simulink model "ALL_JP360_DBW_V6_5_1103"  (R2022a)
settings: Solver=FixedStepAuto  StartTime=0.0  StopTime=inf  FixedStep=0.01  RelTol=1e-3  EnableMultiTasking=on
model workspace (MAT data in the model file):
  g = 9.8
undefined symbols (not defined in the file or in its folder): canChannel, delta_v_p, IPM_Line_C0, IPM_Line_C1, IPM_Line_C2, IPM_Line_C3, M, M_p, MRR_ObjDistX, MRR_ObjDistY, MRR_ObjFusionCamID, MRR_ObjFusionSig, MRR_ObjID, MRR_ObjRelVelX, MRR_ObjRelVelY, MRR_ObjType, MRR_ObjUpdFlg, none, obj_vaild, untracktime, V, videoinput
libraries: canfdmsglib x230, canfdlib x76, slpidlib x24, simulink x18, dspstat3 x14, ctrlSharedLib x1, simulink_extras x1, imaqlib x1, realtime_pacer_lib x1, dspvision x1, visionsinks x1
(part 29 of 55)

== system ALL_JP360_DBW_V6_5_1103/MsgFromCAN/SRR_ADCU_MsgFromCAN/SRR_ADCU_RLR_Freespace_0x1F4 ==
  SRR_ADCU_RLR_Freespace_0x1F4FromInData : Inport  OutDataTypeStr=Bus:CAN_FD_MESSAGE_BUS
  Bus Creator : BusCreator  Inputs=56  OutDataTypeStr=Bus:SRR_ADCU_RLR_Freespace_0x1F4  NonVirtualBus=on
  CAN FD Unpack : canfdmsglib/CAN FD Unpack  CANdbFile=V363 SRR Private CAN-V1.3.dbc  MsgList=(none)  MsgName=RLR_Freespace_0x1F4  ProtocolMode=CAN FD  MsgIDType=Standard (11-bit identifier)  MsgIdentifier=500  MsgLength=64  SignalInfo={'RLR_CRCCheck_FSP_MSG4','504','16','BE','unsigned','Standard','0','1','0','0','65535';'RLR_FreespaceSectorConfidence103','12','2','BE','unsigned','Standard','0','1','0','0','3';'RLR_FreespaceSectorConfidence104','30','2','BE','unsigned','Standard','0','1','0','0','3';'RLR_FreespaceSectorConfidence105','32','2','BE','unsigned','Standard','0','1','0','0','3';'RLR_FreespaceSectorConfidence106','50','2','BE','unsigned','Standard','0','1','0','0','3';'RLR_FreespaceSectorConfidence107','68','2','BE','unsigned','Standard','0','1','0','0','3';'RLR_FreespaceSectorConfidence108','86','2','BE','unsigned','Standard','0','1','0','0','3';'RLR_FreespaceSectorConfidence109','88','2','BE','unsigned','Standard','0','1','0','0','3';'RLR_FreespaceSectorConfidence110','106','2','BE','unsigned','Standard','0','1','0','0','3';'RLR_FreespaceSectorConfidence111','124','2','BE','unsigned','Standard','0','1','0','0','3';'RLR_FreespaceSectorConfidence112','142','2','BE','unsigned','Standard','0','1','0','0','3';'RLR_FreespaceSectorConfidence113','144','2','BE','unsigned','Standard','0','1','0','0','3';'RLR_FreespaceSectorConfidence114','162','2','BE','unsigned','Standard','0','1','0','0','3';'RLR_FreespaceSectorConfidence115','180','2','BE','unsigned','Standard','0','1','0','0','3';'RLR_FreespaceSectorConfidence116','198','2','BE','unsigned','Standard','0','1','0','0','3';'RLR_FreespaceSectorConfidence117','200','2','BE','unsigned','Standard','0','1','0','0','3';'RLR_FreespaceSectorConfidence118','218','2','BE','unsigned','Standard','0','1','0','0','3';'RLR_FreespaceSectorConfidence119','236','2','BE','unsigned','Standard','0','1','0','0','3';'RLR_FreespaceSectorConfidence120','254','2','BE','unsigned','Standard','0','1','0','0','3';'RLR_FreespaceSectorDistance103','14','10','BE','unsigned','Standard','0','0.1','0','0','100';'RLR_FreespaceSectorDistance104','16','10','BE','unsigned','Standard','0','0.1','0','0','100';'RLR_FreespaceSectorDistance105','34','10','BE','unsigned','Standard','0','0.1','0','0','100';'RLR_FreespaceSectorDistance106','52','10','BE','unsigned','Standard','0','0.1','0','0','100';'RLR_FreespaceSectorDistance107','70','10','BE','unsigned','Standard','0','0.1','0','0','100';'RLR_FreespaceSectorDistance108','72','10','BE','unsigned','Standard','0','0.1','0','0','100';'RLR_FreespaceSectorDistance109','90','10','BE','unsigned','Standard','0','0.1','0','0','100';'RLR_FreespaceSectorDistance110','108','10','BE','unsigned','Standard','0','0.1','0','0','100';'RLR_FreespaceSectorDistance111','126','10','BE','unsigned','Standard','0','0.1','0','0','100';'RLR_FreespaceSectorDistance112','128','10','BE','unsigned','Standard','0','0.1','0','0','100';'RLR_FreespaceSectorDistance113','146','10','BE','unsigned','Standard','0','0.1','0','0','100';'RLR_FreespaceSectorDistance114','164','10','BE','unsigned','Standard','0','0.1','0','0','100';'RLR_FreespaceSectorDistance115','182','10','BE','unsigned','Standard','0','0.1','0','0','100';'RLR_FreespaceSectorDistance116','184','10','BE','unsigned','Standard','0','0.1','0','0','100';'RLR_FreespaceSectorDistance117','202','10','BE','unsigned','Standard','0','0.1','0','0','100';'RLR_FreespaceSectorDistance118','220','10','BE','unsigned','Standard','0','0.1','0','0','100';'RLR_FreespaceSectorDistance119','238','10','BE','unsigned','Standard','0','0.1','0','0','100';'RLR_FreespaceSectorDistance120','240','10','BE','unsigned','Standard','0','0.1','0','0','100';'RLR_FreespaceSectorKinestate103','10','2','BE','unsigned','Standard','0','1','0','0','3';'RLR_FreespaceSectorKinestate104','28','2','BE','unsigned','Standard','0','1','0','0','3';'RLR_FreespaceSectorKinestate105','46','2','BE','unsigned','Standard','0','1','0','0','3';'RLR_FreespaceSectorKinestate106','48','2','BE','unsigned','Standard','0','1','0','0','3';'RLR_FreespaceSectorKinestate107','66','2','BE','unsigned','Standard','0','1','0','0','3';'RLR_FreespaceSectorKinestate108','84','2','BE','unsigned','Standard','0','1','0','0','3';'RLR_FreespaceSectorKinestate109','102','2','BE','unsigned','Standard','0','1','0','0','3';'RLR_FreespaceSectorKinestate110','104','2','BE','unsigned','Standard','0','1','0','0','3';'RLR_FreespaceSectorKinestate111','122','2','BE','unsigned','Standard','0','1','0','0','3';'RLR_FreespaceSectorKinestate112','140','2','BE','unsigned','Standard','0','1','0','0','3';'RLR_FreespaceSectorKinestate113','158','2','BE','unsigned','Standard','0','1','0','0','3';'RLR_FreespaceSectorKinestate114','160','2','BE','unsigned','Standard','0','1','0','0','3';'RLR_FreespaceSectorKinestate115','178','2','BE','unsigned','Standard','0','1','0','0','3';'RLR_FreespaceSectorKinestate116','196','2','BE','unsigned','Standard','0','1','0','0','3';'RLR_FreespaceSectorKinestate117','214','2','BE','unsigned','Standard','0','1','0','0','3';'RLR_FreespaceSectorKinestate118','216','2','BE','unsigned','Standard','0','1','0','0','3';'RLR_FreespaceSectorKinestate119','234','2','BE','unsigned','Standard','0','1','0','0','3';'RLR_FreespaceSectorKinestate120','252','2','BE','unsigned','Standard','0','1','0','0','3';'RLR_RollingCounter_FSP_MSG4','488','4','BE','unsigned','Standard','0','1','0','0','15'}  IDPort=off  TimestampPort=off  ErrorPort=off  RemotePort=off  LengthPort=off  StatusPort=off  BRSPort=off  ESIPort=off  DLCPort=off  ApplyMinMax=off
      settings: SourceProductBaseCode=ME,XP,VN  DataFormat=CANdb specified signals
  Data Type Conversion1 : DataTypeConversion  OutDataTypeStr=uint16  SaturateOnIntegerOverflow=off  RndMeth=Floor
  Data Type Conversion{2..19,38..56} (37 alike) : DataTypeConversion  OutDataTypeStr=int8  SaturateOnIntegerOverflow=off  RndMeth=Floor
  Data Type Conversion{20..37} (18 alike) : DataTypeConversion  OutDataTypeStr=single  SaturateOnIntegerOverflow=off  RndMeth=Floor
  SRR_ADCU_RLR_Freespace_0x1F4FromOutData : Outport  OutDataTypeStr=Bus:SRR_ADCU_RLR_Freespace_0x1F4
  wires:
  CAN FD Unpack/1 -> Data Type Conversion1/1
  CAN FD Unpack/2 -> Data Type Conversion2/1
  CAN FD Unpack/3 -> Data Type Conversion3/1
  CAN FD Unpack/4 -> Data Type Conversion4/1
  CAN FD Unpack/5 -> Data Type Conversion5/1
  CAN FD Unpack/6 -> Data Type Conversion6/1
  CAN FD Unpack/7 -> Data Type Conversion7/1
  CAN FD Unpack/8 -> Data Type Conversion8/1
  CAN FD Unpack/9 -> Data Type Conversion9/1
  CAN FD Unpack/10 -> Data Type Conversion10/1
  CAN FD Unpack/11 -> Data Type Conversion11/1
  CAN FD Unpack/12 -> Data Type Conversion12/1
  CAN FD Unpack/13 -> Data Type Conversion13/1
  CAN FD Unpack/14 -> Data Type Conversion14/1
  CAN FD Unpack/15 -> Data Type Conversion15/1
  CAN FD Unpack/16 -> Data Type Conversion16/1
  CAN FD Unpack/17 -> Data Type Conversion17/1
  CAN FD Unpack/18 -> Data Type Conversion18/1
  CAN FD Unpack/19 -> Data Type Conversion19/1
  CAN FD Unpack/20 -> Data Type Conversion20/1
  CAN FD Unpack/21 -> Data Type Conversion21/1
  CAN FD Unpack/22 -> Data Type Conversion22/1
  CAN FD Unpack/23 -> Data Type Conversion23/1
  CAN FD Unpack/24 -> Data Type Conversion24/1
  CAN FD Unpack/25 -> Data Type Conversion25/1
  CAN FD Unpack/26 -> Data Type Conversion26/1
  CAN FD Unpack/27 -> Data Type Conversion27/1
  CAN FD Unpack/28 -> Data Type Conversion28/1
  CAN FD Unpack/29 -> Data Type Conversion29/1
  CAN FD Unpack/30 -> Data Type Conversion30/1
  CAN FD Unpack/31 -> Data Type Conversion31/1
  CAN FD Unpack/32 -> Data Type Conversion32/1
  CAN FD Unpack/33 -> Data Type Conversion33/1
  CAN FD Unpack/34 -> Data Type Conversion34/1
  CAN FD Unpack/35 -> Data Type Conversion35/1
  CAN FD Unpack/36 -> Data Type Conversion36/1
  CAN FD Unpack/37 -> Data Type Conversion37/1
  CAN FD Unpack/38 -> Data Type Conversion38/1
  CAN FD Unpack/39 -> Data Type Conversion39/1
  CAN FD Unpack/40 -> Data Type Conversion40/1
  CAN FD Unpack/41 -> Data Type Conversion41/1
  CAN FD Unpack/42 -> Data Type Conversion42/1
  CAN FD Unpack/43 -> Data Type Conversion43/1
  CAN FD Unpack/44 -> Data Type Conversion44/1
  CAN FD Unpack/45 -> Data Type Conversion45/1
  CAN FD Unpack/46 -> Data Type Conversion46/1
  CAN FD Unpack/47 -> Data Type Conversion47/1
  CAN FD Unpack/48 -> Data Type Conversion48/1
  CAN FD Unpack/49 -> Data Type Conversion49/1
  CAN FD Unpack/50 -> Data Type Conversion50/1
  CAN FD Unpack/51 -> Data Type Conversion51/1
  CAN FD Unpack/52 -> Data Type Conversion52/1
  CAN FD Unpack/53 -> Data Type Conversion53/1
  CAN FD Unpack/54 -> Data Type Conversion54/1
  CAN FD Unpack/55 -> Data Type Conversion55/1
  CAN FD Unpack/56 -> Data Type Conversion56/1
  Data Type Conversion1/1 -> Bus Creator/1  "RLR_CRCCheck_FSP_MSG4"
  Data Type Conversion2/1 -> Bus Creator/2  "RLR_FreespaceSectorConfidence103"
  Data Type Conversion3/1 -> Bus Creator/3  "RLR_FreespaceSectorConfidence104"
  Data Type Conversion4/1 -> Bus Creator/4  "RLR_FreespaceSectorConfidence105"
  Data Type Conversion5/1 -> Bus Creator/5  "RLR_FreespaceSectorConfidence106"
  Data Type Conversion6/1 -> Bus Creator/6  "RLR_FreespaceSectorConfidence107"
  Data Type Conversion7/1 -> Bus Creator/7  "RLR_FreespaceSectorConfidence108"
  Data Type Conversion8/1 -> Bus Creator/8  "RLR_FreespaceSectorConfidence109"
  Data Type Conversion9/1 -> Bus Creator/9  "RLR_FreespaceSectorConfidence110"
  Data Type Conversion10/1 -> Bus Creator/10  "RLR_FreespaceSectorConfidence111"
  Data Type Conversion11/1 -> Bus Creator/11  "RLR_FreespaceSectorConfidence112"
  Data Type Conversion12/1 -> Bus Creator/12  "RLR_FreespaceSectorConfidence113"
  Data Type Conversion13/1 -> Bus Creator/13  "RLR_FreespaceSectorConfidence114"
  Data Type Conversion14/1 -> Bus Creator/14  "RLR_FreespaceSectorConfidence115"
  Data Type Conversion15/1 -> Bus Creator/15  "RLR_FreespaceSectorConfidence116"
  Data Type Conversion16/1 -> Bus Creator/16  "RLR_FreespaceSectorConfidence117"
  Data Type Conversion17/1 -> Bus Creator/17  "RLR_FreespaceSectorConfidence118"
  Data Type Conversion18/1 -> Bus Creator/18  "RLR_FreespaceSectorConfidence119"
  Data Type Conversion19/1 -> Bus Creator/19  "RLR_FreespaceSectorConfidence120"
  Data Type Conversion20/1 -> Bus Creator/20  "RLR_FreespaceSectorDistance103"
  Data Type Conversion21/1 -> Bus Creator/21  "RLR_FreespaceSectorDistance104"
  Data Type Conversion22/1 -> Bus Creator/22  "RLR_FreespaceSectorDistance105"
  Data Type Conversion23/1 -> Bus Creator/23  "RLR_FreespaceSectorDistance106"
  Data Type Conversion24/1 -> Bus Creator/24  "RLR_FreespaceSectorDistance107"
  Data Type Conversion25/1 -> Bus Creator/25  "RLR_FreespaceSectorDistance108"
  Data Type Conversion26/1 -> Bus Creator/26  "RLR_FreespaceSectorDistance109"
  Data Type Conversion27/1 -> Bus Creator/27  "RLR_FreespaceSectorDistance110"
  Data Type Conversion28/1 -> Bus Creator/28  "RLR_FreespaceSectorDistance111"
  Data Type Conversion29/1 -> Bus Creator/29  "RLR_FreespaceSectorDistance112"
  Data Type Conversion30/1 -> Bus Creator/30  "RLR_FreespaceSectorDistance113"
  Data Type Conversion31/1 -> Bus Creator/31  "RLR_FreespaceSectorDistance114"
  Data Type Conversion32/1 -> Bus Creator/32  "RLR_FreespaceSectorDistance115"
  Data Type Conversion33/1 -> Bus Creator/33  "RLR_FreespaceSectorDistance116"
  Data Type Conversion34/1 -> Bus Creator/34  "RLR_FreespaceSectorDistance117"
  Data Type Conversion35/1 -> Bus Creator/35  "RLR_FreespaceSectorDistance118"
  Data Type Conversion36/1 -> Bus Creator/36  "RLR_FreespaceSectorDistance119"
  Data Type Conversion37/1 -> Bus Creator/37  "RLR_FreespaceSectorDistance120"
  Data Type Conversion38/1 -> Bus Creator/38  "RLR_FreespaceSectorKinestate103"
  Data Type Conversion39/1 -> Bus Creator/39  "RLR_FreespaceSectorKinestate104"
  Data Type Conversion40/1 -> Bus Creator/40  "RLR_FreespaceSectorKinestate105"
  Data Type Conversion41/1 -> Bus Creator/41  "RLR_FreespaceSectorKinestate106"
  Data Type Conversion42/1 -> Bus Creator/42  "RLR_FreespaceSectorKinestate107"
  Data Type Conversion43/1 -> Bus Creator/43  "RLR_FreespaceSectorKinestate108"
  Data Type Conversion44/1 -> Bus Creator/44  "RLR_FreespaceSectorKinestate109"
  Data Type Conversion45/1 -> Bus Creator/45  "RLR_FreespaceSectorKinestate110"
  Data Type Conversion46/1 -> Bus Creator/46  "RLR_FreespaceSectorKinestate111"
  Data Type Conversion47/1 -> Bus Creator/47  "RLR_FreespaceSectorKinestate112"
  Data Type Conversion48/1 -> Bus Creator/48  "RLR_FreespaceSectorKinestate113"
  Data Type Conversion49/1 -> Bus Creator/49  "RLR_FreespaceSectorKinestate114"
  Data Type Conversion50/1 -> Bus Creator/50  "RLR_FreespaceSectorKinestate115"
  Data Type Conversion51/1 -> Bus Creator/51  "RLR_FreespaceSectorKinestate116"
  Data Type Conversion52/1 -> Bus Creator/52  "RLR_FreespaceSectorKinestate117"
  Data Type Conversion53/1 -> Bus Creator/53  "RLR_FreespaceSectorKinestate118"
  Data Type Conversion54/1 -> Bus Creator/54  "RLR_FreespaceSectorKinestate119"
  Data Type Conversion55/1 -> Bus Creator/55  "RLR_FreespaceSectorKinestate120"
  Data Type Conversion56/1 -> Bus Creator/56  "RLR_RollingCounter_FSP_MSG4"
  Bus Creator/1 -> SRR_ADCU_RLR_Freespace_0x1F4FromOutData/1  "SRR_ADCU_RLR_Freespace_0x1F4FromOutData"
  SRR_ADCU_RLR_Freespace_0x1F4FromInData/1 -> CAN FD Unpack/1  "SRR_ADCU_RLR_Freespace_0x1F4FromInData"

== system ALL_JP360_DBW_V6_5_1103/MsgFromCAN/SRR_ADCU_MsgFromCAN/SRR_ADCU_RLR_OBJPos10_0x1CD ==
  SRR_ADCU_RLR_OBJPos10_0x1CDFromInData : Inport  OutDataTypeStr=Bus:CAN_FD_MESSAGE_BUS
  Bus Creator : BusCreator  Inputs=42  OutDataTypeStr=Bus:SRR_ADCU_RLR_OBJPos10_0x1CD  NonVirtualBus=on
  CAN FD Unpack : canfdmsglib/CAN FD Unpack  CANdbFile=V363 SRR Private CAN-V1.3.dbc  MsgList=(none)  MsgName=RLR_OBJPos10_0x1CD  ProtocolMode=CAN FD  MsgIDType=Standard (11-bit identifier)  MsgIdentifier=461  MsgLength=48  SignalInfo={'RLR_CRCCheck_0x1CD','376','16','BE','unsigned','Standard','0','1','0','0','65535';'RLR_OBJ19_Dx','79','13','BE','unsigned','Standard','0','0.0625','-256','-256','255.938';'RLR_OBJ19_Dy','60','11','BE','unsigned','Standard','0','0.125','-128','-128','127.875';'RLR_OBJ19_ExistProb','112','6','BE','unsigned','Standard','0','2','0','0','100';'RLR_OBJ19_HeadingAngle','55','10','BE','unsigned','Standard','0','0.01','-3.14','-3.14','3.14';'RLR_OBJ19_Height','26','9','BE','unsigned','Standard','0','0.01','0','0','5.11';'RLR_OBJ19_Length','33','9','BE','unsigned','Standard','0','0.05','0','0','25.5';'RLR_OBJ19_Measured','126','2','BE','unsigned','Standard','0','1','0','0','3';'RLR_OBJ19_Motion_Status','162','3','BE','unsigned','Standard','0','1','0','0','7';'RLR_OBJ19_ObstacleProb','120','6','BE','unsigned','Standard','0','2','0','0','100';'RLR_OBJ19_RefPointDx','144','13','BE','unsigned','Standard','0','0.0625','-256','-256','255.938';'RLR_OBJ19_RefPointDy','141','11','BE','unsigned','Standard','0','0.125','-128','-128','127.875';'RLR_OBJ19_RefPointLoc','157','3','BE','unsigned','Standard','0','1','0','0','7';'RLR_OBJ19_RelAx','118','9','BE','unsigned','Standard','0','0.0625','-16','-16','15.9375';'RLR_OBJ19_RelAy','111','10','BE','unsigned','Standard','0','0.03125','-16','-16','15.9688';'RLR_OBJ19_RelVx','89','12','BE','unsigned','Standard','0','0.0625','-128','-128','127.938';'RLR_OBJ19_RelVy','85','10','BE','unsigned','Standard','0','0.125','-64','-64','63.875';'RLR_OBJ19_Track_Age','165','8','BE','unsigned','Standard','0','1','0','0','255';'RLR_OBJ19_Track_ID','1','7','BE','unsigned','Standard','0','1','0','0','127';'RLR_OBJ19_Type','14','3','BE','unsigned','Standard','0','1','0','0','7';'RLR_OBJ19_Width','19','11','BE','unsigned','Standard','0','0.01','0','0','12';'RLR_OBJ20_Dx','247','13','BE','unsigned','Standard','0','0.0625','-256','-256','255.938';'RLR_OBJ20_Dy','228','11','BE','unsigned','Standard','0','0.125','-128','-128','127.875';'RLR_OBJ20_ExistProb','280','6','BE','unsigned','Standard','0','2','0','0','100';'RLR_OBJ20_HeadingAngle','223','10','BE','unsigned','Standard','0','0.01','-3.14','-3.14','3.14';'RLR_OBJ20_Height','194','9','BE','unsigned','Standard','0','0.01','0','0','5.11';'RLR_OBJ20_Length','201','9','BE','unsigned','Standard','0','0.05','0','0','25.5';'RLR_OBJ20_Measured','294','2','BE','unsigned','Standard','0','1','0','0','3';'RLR_OBJ20_Motion_Status','330','3','BE','unsigned','Standard','0','1','0','0','7';'RLR_OBJ20_ObstacleProb','288','6','BE','unsigned','Standard','0','2','0','0','100';'RLR_OBJ20_RefPointDx','312','13','BE','unsigned','Standard','0','0.0625','-256','-256','255.938';'RLR_OBJ20_RefPointDy','309','11','BE','unsigned','Standard','0','0.125','-128','-128','127.875';'RLR_OBJ20_RefPointLoc','325','3','BE','unsigned','Standard','0','1','0','0','7';'RLR_OBJ20_RelAx','286','9','BE','unsigned','Standard','0','0.0625','-16','-16','15.9375';'RLR_OBJ20_RelAy','279','10','BE','unsigned','Standard','0','0.03125','-16','-16','15.9688';'RLR_OBJ20_RelVx','257','12','BE','unsigned','Standard','0','0.0625','-128','-128','127.938';'RLR_OBJ20_RelVy','253','10','BE','unsigned','Standard','0','0.125','-64','-64','63.875';'RLR_OBJ20_Track_Age','333','8','BE','unsigned','Standard','0','1','0','0','255';'RLR_OBJ20_Track_ID','169','7','BE','unsigned','Standard','0','1','0','0','127';'RLR_OBJ20_Type','182','3','BE','unsigned','Standard','0','1','0','0','7';'RLR_OBJ20_Width','187','11','BE','unsigned','Standard','0','0.01','0','0','12';'RLR_RollingCounter_0x1CD','360','4','BE','unsigned','Standard','0','1','0','0','15'}  IDPort=off  TimestampPort=off  ErrorPort=off  RemotePort=off  LengthPort=off  StatusPort=off  BRSPort=off  ESIPort=off  DLCPort=off  ApplyMinMax=off
      settings: SourceProductBaseCode=ME,XP,VN  DataFormat=CANdb specified signals
  Data Type Conversion1 : DataTypeConversion  OutDataTypeStr=uint16  SaturateOnIntegerOverflow=off  RndMeth=Floor
  Data Type Conversion{4,8..10,13,19..20,24,28..30,33,39..40,42} (15 alike) : DataTypeConversion  OutDataTypeStr=int8  SaturateOnIntegerOverflow=off  RndMeth=Floor
  Data Type Conversion{2..3,5..7,11..12,14..17,21..23,25..27,31..32,34..37,41} (24 alike) : DataTypeConversion  OutDataTypeStr=single  SaturateOnIntegerOverflow=off  RndMeth=Floor
  Data Type Conversion18 : DataTypeConversion  OutDataTypeStr=uint8  SaturateOnIntegerOverflow=off  RndMeth=Floor
  Data Type Conversion38 : DataTypeConversion  OutDataTypeStr=uint8  SaturateOnIntegerOverflow=off  RndMeth=Floor
  SRR_ADCU_RLR_OBJPos10_0x1CDFromOutData : Outport  OutDataTypeStr=Bus:SRR_ADCU_RLR_OBJPos10_0x1CD
  wires:
  CAN FD Unpack/1 -> Data Type Conversion1/1
  CAN FD Unpack/2 -> Data Type Conversion2/1
  CAN FD Unpack/3 -> Data Type Conversion3/1
  CAN FD Unpack/4 -> Data Type Conversion4/1
  CAN FD Unpack/5 -> Data Type Conversion5/1
  CAN FD Unpack/6 -> Data Type Conversion6/1
  CAN FD Unpack/7 -> Data Type Conversion7/1
  CAN FD Unpack/8 -> Data Type Conversion8/1
  CAN FD Unpack/9 -> Data Type Conversion9/1
  CAN FD Unpack/10 -> Data Type Conversion10/1
  CAN FD Unpack/11 -> Data Type Conversion11/1
  CAN FD Unpack/12 -> Data Type Conversion12/1
  CAN FD Unpack/13 -> Data Type Conversion13/1
  CAN FD Unpack/14 -> Data Type Conversion14/1
  CAN FD Unpack/15 -> Data Type Conversion15/1
  CAN FD Unpack/16 -> Data Type Conversion16/1
  CAN FD Unpack/17 -> Data Type Conversion17/1
  CAN FD Unpack/18 -> Data Type Conversion18/1
  CAN FD Unpack/19 -> Data Type Conversion19/1
  CAN FD Unpack/20 -> Data Type Conversion20/1
  CAN FD Unpack/21 -> Data Type Conversion21/1
  CAN FD Unpack/22 -> Data Type Conversion22/1
  CAN FD Unpack/23 -> Data Type Conversion23/1
  CAN FD Unpack/24 -> Data Type Conversion24/1
  CAN FD Unpack/25 -> Data Type Conversion25/1
  CAN FD Unpack/26 -> Data Type Conversion26/1
  CAN FD Unpack/27 -> Data Type Conversion27/1
  CAN FD Unpack/28 -> Data Type Conversion28/1
  CAN FD Unpack/29 -> Data Type Conversion29/1
  CAN FD Unpack/30 -> Data Type Conversion30/1
  CAN FD Unpack/31 -> Data Type Conversion31/1
  CAN FD Unpack/32 -> Data Type Conversion32/1
  CAN FD Unpack/33 -> Data Type Conversion33/1
  CAN FD Unpack/34 -> Data Type Conversion34/1
  CAN FD Unpack/35 -> Data Type Conversion35/1
  CAN FD Unpack/36 -> Data Type Conversion36/1
  CAN FD Unpack/37 -> Data Type Conversion37/1
  CAN FD Unpack/38 -> Data Type Conversion38/1
  CAN FD Unpack/39 -> Data Type Conversion39/1
  CAN FD Unpack/40 -> Data Type Conversion40/1
  CAN FD Unpack/41 -> Data Type Conversion41/1
  CAN FD Unpack/42 -> Data Type Conversion42/1
  Data Type Conversion1/1 -> Bus Creator/1  "RLR_CRCCheck_0x1CD"
  Data Type Conversion2/1 -> Bus Creator/2  "RLR_OBJ19_Dx"
  Data Type Conversion3/1 -> Bus Creator/3  "RLR_OBJ19_Dy"
  Data Type Conversion4/1 -> Bus Creator/4  "RLR_OBJ19_ExistProb"
  Data Type Conversion5/1 -> Bus Creator/5  "RLR_OBJ19_HeadingAngle"
  Data Type Conversion6/1 -> Bus Creator/6  "RLR_OBJ19_Height"
  Data Type Conversion7/1 -> Bus Creator/7  "RLR_OBJ19_Length"
  Data Type Conversion8/1 -> Bus Creator/8  "RLR_OBJ19_Measured"
  Data Type Conversion9/1 -> Bus Creator/9  "RLR_OBJ19_Motion_Status"
  Data Type Conversion10/1 -> Bus Creator/10  "RLR_OBJ19_ObstacleProb"
  Data Type Conversion11/1 -> Bus Creator/11  "RLR_OBJ19_RefPointDx"
  Data Type Conversion12/1 -> Bus Creator/12  "RLR_OBJ19_RefPointDy"
  Data Type Conversion13/1 -> Bus Creator/13  "RLR_OBJ19_RefPointLoc"
  Data Type Conversion14/1 -> Bus Creator/14  "RLR_OBJ19_RelAx"
  Data Type Conversion15/1 -> Bus Creator/15  "RLR_OBJ19_RelAy"
  Data Type Conversion16/1 -> Bus Creator/16  "RLR_OBJ19_RelVx"
  Data Type Conversion17/1 -> Bus Creator/17  "RLR_OBJ19_RelVy"
  Data Type Conversion18/1 -> Bus Creator/18  "RLR_OBJ19_Track_Age"
  Data Type Conversion19/1 -> Bus Creator/19  "RLR_OBJ19_Track_ID"
  Data Type Conversion20/1 -> Bus Creator/20  "RLR_OBJ19_Type"
  Data Type Conversion21/1 -> Bus Creator/21  "RLR_OBJ19_Width"
  Data Type Conversion22/1 -> Bus Creator/22  "RLR_OBJ20_Dx"
  Data Type Conversion23/1 -> Bus Creator/23  "RLR_OBJ20_Dy"
  Data Type Conversion24/1 -> Bus Creator/24  "RLR_OBJ20_ExistProb"
  Data Type Conversion25/1 -> Bus Creator/25  "RLR_OBJ20_HeadingAngle"
  Data Type Conversion26/1 -> Bus Creator/26  "RLR_OBJ20_Height"
  Data Type Conversion27/1 -> Bus Creator/27  "RLR_OBJ20_Length"
  Data Type Conversion28/1 -> Bus Creator/28  "RLR_OBJ20_Measured"
  Data Type Conversion29/1 -> Bus Creator/29  "RLR_OBJ20_Motion_Status"
  Data Type Conversion30/1 -> Bus Creator/30  "RLR_OBJ20_ObstacleProb"
  Data Type Conversion31/1 -> Bus Creator/31  "RLR_OBJ20_RefPointDx"
  Data Type Conversion32/1 -> Bus Creator/32  "RLR_OBJ20_RefPointDy"
  Data Type Conversion33/1 -> Bus Creator/33  "RLR_OBJ20_RefPointLoc"
  Data Type Conversion34/1 -> Bus Creator/34  "RLR_OBJ20_RelAx"
  Data Type Conversion35/1 -> Bus Creator/35  "RLR_OBJ20_RelAy"
  Data Type Conversion36/1 -> Bus Creator/36  "RLR_OBJ20_RelVx"
  Data Type Conversion37/1 -> Bus Creator/37  "RLR_OBJ20_RelVy"
  Data Type Conversion38/1 -> Bus Creator/38  "RLR_OBJ20_Track_Age"
  Data Type Conversion39/1 -> Bus Creator/39  "RLR_OBJ20_Track_ID"
  Data Type Conversion40/1 -> Bus Creator/40  "RLR_OBJ20_Type"
  Data Type Conversion41/1 -> Bus Creator/41  "RLR_OBJ20_Width"
  Data Type Conversion42/1 -> Bus Creator/42  "RLR_RollingCounter_0x1CD"
  Bus Creator/1 -> SRR_ADCU_RLR_OBJPos10_0x1CDFromOutData/1  "SRR_ADCU_RLR_OBJPos10_0x1CDFromOutData"
  SRR_ADCU_RLR_OBJPos10_0x1CDFromInData/1 -> CAN FD Unpack/1  "SRR_ADCU_RLR_OBJPos10_0x1CDFromInData"

== system ALL_JP360_DBW_V6_5_1103/MsgFromCAN/SRR_ADCU_MsgFromCAN/SRR_ADCU_RLR_OBJPos11_0x1CE ==
  SRR_ADCU_RLR_OBJPos11_0x1CEFromInData : Inport  OutDataTypeStr=Bus:CAN_FD_MESSAGE_BUS
  Bus Creator : BusCreator  Inputs=42  OutDataTypeStr=Bus:SRR_ADCU_RLR_OBJPos11_0x1CE  NonVirtualBus=on
  CAN FD Unpack : canfdmsglib/CAN FD Unpack  CANdbFile=V363 SRR Private CAN-V1.3.dbc  MsgList=(none)  MsgName=RLR_OBJPos11_0x1CE  ProtocolMode=CAN FD  MsgIDType=Standard (11-bit identifier)  MsgIdentifier=462  MsgLength=48  SignalInfo={'RLR_CRCCheck_0x1CE','376','16','BE','unsigned','Standard','0','1','0','0','65535';'RLR_OBJ21_Dx','79','13','BE','unsigned','Standard','0','0.0625','-256','-256','255.938';'RLR_OBJ21_Dy','60','11','BE','unsigned','Standard','0','0.125','-128','-128','127.875';'RLR_OBJ21_ExistProb','112','6','BE','unsigned','Standard','0','2','0','0','100';'RLR_OBJ21_HeadingAngle','55','10','BE','unsigned','Standard','0','0.01','-3.14','-3.14','3.14';'RLR_OBJ21_Height','26','9','BE','unsigned','Standard','0','0.01','0','0','5.11';'RLR_OBJ21_Length','33','9','BE','unsigned','Standard','0','0.05','0','0','25.5';'RLR_OBJ21_Measured','126','2','BE','unsigned','Standard','0','1','0','0','3';'RLR_OBJ21_Motion_Status','162','3','BE','unsigned','Standard','0','1','0','0','7';'RLR_OBJ21_ObstacleProb','120','6','BE','unsigned','Standard','0','2','0','0','100';'RLR_OBJ21_RefPointDx','144','13','BE','unsigned','Standard','0','0.0625','-256','-256','255.938';'RLR_OBJ21_RefPointDy','141','11','BE','unsigned','Standard','0','0.125','-128','-128','127.875';'RLR_OBJ21_RefPointLoc','157','3','BE','unsigned','Standard','0','1','0','0','7';'RLR_OBJ21_RelAx','118','9','BE','unsigned','Standard','0','0.0625','-16','-16','15.9375';'RLR_OBJ21_RelAy','111','10','BE','unsigned','Standard','0','0.03125','-16','-16','15.9688';'RLR_OBJ21_RelVx','89','12','BE','unsigned','Standard','0','0.0625','-128','-128','127.938';'RLR_OBJ21_RelVy','85','10','BE','unsigned','Standard','0','0.125','-64','-64','63.875';'RLR_OBJ21_Track_Age','165','8','BE','unsigned','Standard','0','1','0','0','255';'RLR_OBJ21_Track_ID','1','7','BE','unsigned','Standard','0','1','0','0','127';'RLR_OBJ21_Type','14','3','BE','unsigned','Standard','0','1','0','0','7';'RLR_OBJ21_Width','19','11','BE','unsigned','Standard','0','0.01','0','0','12';'RLR_OBJ22_Dx','247','13','BE','unsigned','Standard','0','0.0625','-256','-256','255.938';'RLR_OBJ22_Dy','228','11','BE','unsigned','Standard','0','0.125','-128','-128','127.875';'RLR_OBJ22_ExistProb','280','6','BE','unsigned','Standard','0','2','0','0','100';'RLR_OBJ22_HeadingAngle','223','10','BE','unsigned','Standard','0','0.01','-3.14','-3.14','3.14';'RLR_OBJ22_Height','194','9','BE','unsigned','Standard','0','0.01','0','0','5.11';'RLR_OBJ22_Length','201','9','BE','unsigned','Standard','0','0.05','0','0','25.5';'RLR_OBJ22_Measured','294','2','BE','unsigned','Standard','0','1','0','0','3';'RLR_OBJ22_Motion_Status','330','3','BE','unsigned','Standard','0','1','0','0','7';'RLR_OBJ22_ObstacleProb','288','6','BE','unsigned','Standard','0','2','0','0','100';'RLR_OBJ22_RefPointDx','312','13','BE','unsigned','Standard','0','0.0625','-256','-256','255.938';'RLR_OBJ22_RefPointDy','309','11','BE','unsigned','Standard','0','0.125','-128','-128','127.875';'RLR_OBJ22_RefPointLoc','325','3','BE','unsigned','Standard','0','1','0','0','7';'RLR_OBJ22_RelAx','286','9','BE','unsigned','Standard','0','0.0625','-16','-16','15.9375';'RLR_OBJ22_RelAy','279','10','BE','unsigned','Standard','0','0.03125','-16','-16','15.9688';'RLR_OBJ22_RelVx','257','12','BE','unsigned','Standard','0','0.0625','-128','-128','127.938';'RLR_OBJ22_RelVy','253','10','BE','unsigned','Standard','0','0.125','-64','-64','63.875';'RLR_OBJ22_Track_Age','333','8','BE','unsigned','Standard','0','1','0','0','255';'RLR_OBJ22_Track_ID','169','7','BE','unsigned','Standard','0','1','0','0','127';'RLR_OBJ22_Type','182','3','BE','unsigned','Standard','0','1','0','0','7';'RLR_OBJ22_Width','187','11','BE','unsigned','Standard','0','0.01','0','0','12';'RLR_RollingCounter_0x1CE','360','4','BE','unsigned','Standard','0','1','0','0','15'}  IDPort=off  TimestampPort=off  ErrorPort=off  RemotePort=off  LengthPort=off  StatusPort=off  BRSPort=off  ESIPort=off  DLCPort=off  ApplyMinMax=off
      settings: SourceProductBaseCode=ME,XP,VN  DataFormat=CANdb specified signals
  Data Type Conversion1 : DataTypeConversion  OutDataTypeStr=uint16  SaturateOnIntegerOverflow=off  RndMeth=Floor
  Data Type Conversion{4,8..10,13,19..20,24,28..30,33,39..40,42} (15 alike) : DataTypeConversion  OutDataTypeStr=int8  SaturateOnIntegerOverflow=off  RndMeth=Floor
  Data Type Conversion{2..3,5..7,11..12,14..17,21..23,25..27,31..32,34..37,41} (24 alike) : DataTypeConversion  OutDataTypeStr=single  SaturateOnIntegerOverflow=off  RndMeth=Floor
  Data Type Conversion18 : DataTypeConversion  OutDataTypeStr=uint8  SaturateOnIntegerOverflow=off  RndMeth=Floor
  Data Type Conversion38 : DataTypeConversion  OutDataTypeStr=uint8  SaturateOnIntegerOverflow=off  RndMeth=Floor
  SRR_ADCU_RLR_OBJPos11_0x1CEFromOutData : Outport  OutDataTypeStr=Bus:SRR_ADCU_RLR_OBJPos11_0x1CE
  wires:
  CAN FD Unpack/1 -> Data Type Conversion1/1
  CAN FD Unpack/2 -> Data Type Conversion2/1
  CAN FD Unpack/3 -> Data Type Conversion3/1
  CAN FD Unpack/4 -> Data Type Conversion4/1
  CAN FD Unpack/5 -> Data Type Conversion5/1
  CAN FD Unpack/6 -> Data Type Conversion6/1
  CAN FD Unpack/7 -> Data Type Conversion7/1
  CAN FD Unpack/8 -> Data Type Conversion8/1
  CAN FD Unpack/9 -> Data Type Conversion9/1
  CAN FD Unpack/10 -> Data Type Conversion10/1
  CAN FD Unpack/11 -> Data Type Conversion11/1
  CAN FD Unpack/12 -> Data Type Conversion12/1
  CAN FD Unpack/13 -> Data Type Conversion13/1
  CAN FD Unpack/14 -> Data Type Conversion14/1
  CAN FD Unpack/15 -> Data Type Conversion15/1
  CAN FD Unpack/16 -> Data Type Conversion16/1
  CAN FD Unpack/17 -> Data Type Conversion17/1
  CAN FD Unpack/18 -> Data Type Conversion18/1
  CAN FD Unpack/19 -> Data Type Conversion19/1
  CAN FD Unpack/20 -> Data Type Conversion20/1
  CAN FD Unpack/21 -> Data Type Conversion21/1
  CAN FD Unpack/22 -> Data Type Conversion22/1
  CAN FD Unpack/23 -> Data Type Conversion23/1
  CAN FD Unpack/24 -> Data Type Conversion24/1
  CAN FD Unpack/25 -> Data Type Conversion25/1
  CAN FD Unpack/26 -> Data Type Conversion26/1
  CAN FD Unpack/27 -> Data Type Conversion27/1
  CAN FD Unpack/28 -> Data Type Conversion28/1
  CAN FD Unpack/29 -> Data Type Conversion29/1
  CAN FD Unpack/30 -> Data Type Conversion30/1
  CAN FD Unpack/31 -> Data Type Conversion31/1
  CAN FD Unpack/32 -> Data Type Conversion32/1
  CAN FD Unpack/33 -> Data Type Conversion33/1
  CAN FD Unpack/34 -> Data Type Conversion34/1
  CAN FD Unpack/35 -> Data Type Conversion35/1
  CAN FD Unpack/36 -> Data Type Conversion36/1
  CAN FD Unpack/37 -> Data Type Conversion37/1
  CAN FD Unpack/38 -> Data Type Conversion38/1
  CAN FD Unpack/39 -> Data Type Conversion39/1
  CAN FD Unpack/40 -> Data Type Conversion40/1
  CAN FD Unpack/41 -> Data Type Conversion41/1
  CAN FD Unpack/42 -> Data Type Conversion42/1
  Data Type Conversion1/1 -> Bus Creator/1  "RLR_CRCCheck_0x1CE"
  Data Type Conversion2/1 -> Bus Creator/2  "RLR_OBJ21_Dx"
  Data Type Conversion3/1 -> Bus Creator/3  "RLR_OBJ21_Dy"
  Data Type Conversion4/1 -> Bus Creator/4  "RLR_OBJ21_ExistProb"
  Data Type Conversion5/1 -> Bus Creator/5  "RLR_OBJ21_HeadingAngle"
  Data Type Conversion6/1 -> Bus Creator/6  "RLR_OBJ21_Height"
  Data Type Conversion7/1 -> Bus Creator/7  "RLR_OBJ21_Length"
  Data Type Conversion8/1 -> Bus Creator/8  "RLR_OBJ21_Measured"
  Data Type Conversion9/1 -> Bus Creator/9  "RLR_OBJ21_Motion_Status"
  Data Type Conversion10/1 -> Bus Creator/10  "RLR_OBJ21_ObstacleProb"
  Data Type Conversion11/1 -> Bus Creator/11  "RLR_OBJ21_RefPointDx"
  Data Type Conversion12/1 -> Bus Creator/12  "RLR_OBJ21_RefPointDy"
  Data Type Conversion13/1 -> Bus Creator/13  "RLR_OBJ21_RefPointLoc"
  Data Type Conversion14/1 -> Bus Creator/14  "RLR_OBJ21_RelAx"
  Data Type Conversion15/1 -> Bus Creator/15  "RLR_OBJ21_RelAy"
  Data Type Conversion16/1 -> Bus Creator/16  "RLR_OBJ21_RelVx"
  Data Type Conversion17/1 -> Bus Creator/17  "RLR_OBJ21_RelVy"
  Data Type Conversion18/1 -> Bus Creator/18  "RLR_OBJ21_Track_Age"
  Data Type Conversion19/1 -> Bus Creator/19  "RLR_OBJ21_Track_ID"
  Data Type Conversion20/1 -> Bus Creator/20  "RLR_OBJ21_Type"
  Data Type Conversion21/1 -> Bus Creator/21  "RLR_OBJ21_Width"
  Data Type Conversion22/1 -> Bus Creator/22  "RLR_OBJ22_Dx"
  Data Type Conversion23/1 -> Bus Creator/23  "RLR_OBJ22_Dy"
  Data Type Conversion24/1 -> Bus Creator/24  "RLR_OBJ22_ExistProb"
  Data Type Conversion25/1 -> Bus Creator/25  "RLR_OBJ22_HeadingAngle"
  Data Type Conversion26/1 -> Bus Creator/26  "RLR_OBJ22_Height"
  Data Type Conversion27/1 -> Bus Creator/27  "RLR_OBJ22_Length"
  Data Type Conversion28/1 -> Bus Creator/28  "RLR_OBJ22_Measured"
  Data Type Conversion29/1 -> Bus Creator/29  "RLR_OBJ22_Motion_Status"
  Data Type Conversion30/1 -> Bus Creator/30  "RLR_OBJ22_ObstacleProb"
  Data Type Conversion31/1 -> Bus Creator/31  "RLR_OBJ22_RefPointDx"
  Data Type Conversion32/1 -> Bus Creator/32  "RLR_OBJ22_RefPointDy"
  Data Type Conversion33/1 -> Bus Creator/33  "RLR_OBJ22_RefPointLoc"
  Data Type Conversion34/1 -> Bus Creator/34  "RLR_OBJ22_RelAx"
  Data Type Conversion35/1 -> Bus Creator/35  "RLR_OBJ22_RelAy"
  Data Type Conversion36/1 -> Bus Creator/36  "RLR_OBJ22_RelVx"
  Data Type Conversion37/1 -> Bus Creator/37  "RLR_OBJ22_RelVy"
  Data Type Conversion38/1 -> Bus Creator/38  "RLR_OBJ22_Track_Age"
  Data Type Conversion39/1 -> Bus Creator/39  "RLR_OBJ22_Track_ID"
  Data Type Conversion40/1 -> Bus Creator/40  "RLR_OBJ22_Type"
  Data Type Conversion41/1 -> Bus Creator/41  "RLR_OBJ22_Width"
  Data Type Conversion42/1 -> Bus Creator/42  "RLR_RollingCounter_0x1CE"
  Bus Creator/1 -> SRR_ADCU_RLR_OBJPos11_0x1CEFromOutData/1  "SRR_ADCU_RLR_OBJPos11_0x1CEFromOutData"
  SRR_ADCU_RLR_OBJPos11_0x1CEFromInData/1 -> CAN FD Unpack/1  "SRR_ADCU_RLR_OBJPos11_0x1CEFromInData"

== system ALL_JP360_DBW_V6_5_1103/MsgFromCAN/SRR_ADCU_MsgFromCAN/SRR_ADCU_RLR_OBJPos12_0x1D1 ==
  SRR_ADCU_RLR_OBJPos12_0x1D1FromInData : Inport  OutDataTypeStr=Bus:CAN_FD_MESSAGE_BUS
  Bus Creator : BusCreator  Inputs=42  OutDataTypeStr=Bus:SRR_ADCU_RLR_OBJPos12_0x1D1  NonVirtualBus=on
  CAN FD Unpack : canfdmsglib/CAN FD Unpack  CANdbFile=V363 SRR Private CAN-V1.3.dbc  MsgList=(none)  MsgName=RLR_OBJPos12_0x1D1  ProtocolMode=CAN FD  MsgIDType=Standard (11-bit identifier)  MsgIdentifier=465  MsgLength=48  SignalInfo={'RLR_CRCCheck_0x1D1','376','16','BE','unsigned','Standard','0','1','0','0','65535';'RLR_OBJ23_Dx','79','13','BE','unsigned','Standard','0','0.0625','-256','-256','255.938';'RLR_OBJ23_Dy','60','11','BE','unsigned','Standard','0','0.125','-128','-128','127.875';'RLR_OBJ23_ExistProb','112','6','BE','unsigned','Standard','0','2','0','0','100';'RLR_OBJ23_HeadingAngle','55','10','BE','unsigned','Standard','0','0.01','-3.14','-3.14','3.14';'RLR_OBJ23_Height','26','9','BE','unsigned','Standard','0','0.01','0','0','5.11';'RLR_OBJ23_Length','33','9','BE','unsigned','Standard','0','0.05','0','0','25.5';'RLR_OBJ23_Measured','126','2','BE','unsigned','Standard','0','1','0','0','3';'RLR_OBJ23_Motion_Status','162','3','BE','unsigned','Standard','0','1','0','0','7';'RLR_OBJ23_ObstacleProb','120','6','BE','unsigned','Standard','0','2','0','0','100';'RLR_OBJ23_RefPointDx','144','13','BE','unsigned','Standard','0','0.0625','-256','-256','255.938';'RLR_OBJ23_RefPointDy','141','11','BE','unsigned','Standard','0','0.125','-128','-128','127.875';'RLR_OBJ23_RefPointLoc','157','3','BE','unsigned','Standard','0','1','0','0','7';'RLR_OBJ23_RelAx','118','9','BE','unsigned','Standard','0','0.0625','-16','-16','15.9375';'RLR_OBJ23_RelAy','111','10','BE','unsigned','Standard','0','0.03125','-16','-16','15.9688';'RLR_OBJ23_RelVx','89','12','BE','unsigned','Standard','0','0.0625','-128','-128','127.938';'RLR_OBJ23_RelVy','85','10','BE','unsigned','Standard','0','0.125','-64','-64','63.875';'RLR_OBJ23_Track_Age','165','8','BE','unsigned','Standard','0','1','0','0','255';'RLR_OBJ23_Track_ID','1','7','BE','unsigned','Standard','0','1','0','0','127';'RLR_OBJ23_Type','14','3','BE','unsigned','Standard','0','1','0','0','7';'RLR_OBJ23_Width','19','11','BE','unsigned','Standard','0','0.01','0','0','12';'RLR_OBJ24_Dx','247','13','BE','unsigned','Standard','0','0.0625','-256','-256','255.938';'RLR_OBJ24_Dy','228','11','BE','unsigned','Standard','0','0.125','-128','-128','127.875';'RLR_OBJ24_ExistProb','280','6','BE','unsigned','Standard','0','2','0','0','100';'RLR_OBJ24_HeadingAngle','223','10','BE','unsigned','Standard','0','0.01','-3.14','-3.14','3.14';'RLR_OBJ24_Height','194','9','BE','unsigned','Standard','0','0.01','0','0','5.11';'RLR_OBJ24_Length','201','9','BE','unsigned','Standard','0','0.05','0','0','25.5';'RLR_OBJ24_Measured','294','2','BE','unsigned','Standard','0','1','0','0','3';'RLR_OBJ24_Motion_Status','330','3','BE','unsigned','Standard','0','1','0','0','7';'RLR_OBJ24_ObstacleProb','288','6','BE','unsigned','Standard','0','2','0','0','100';'RLR_OBJ24_RefPointDx','312','13','BE','unsigned','Standard','0','0.0625','-256','-256','255.938';'RLR_OBJ24_RefPointDy','309','11','BE','unsigned','Standard','0','0.125','-128','-128','127.875';'RLR_OBJ24_RefPointLoc','325','3','BE','unsigned','Standard','0','1','0','0','7';'RLR_OBJ24_RelAx','286','9','BE','unsigned','Standard','0','0.0625','-16','-16','15.9375';'RLR_OBJ24_RelAy','279','10','BE','unsigned','Standard','0','0.03125','-16','-16','15.9688';'RLR_OBJ24_RelVx','257','12','BE','unsigned','Standard','0','0.0625','-128','-128','127.938';'RLR_OBJ24_RelVy','253','10','BE','unsigned','Standard','0','0.125','-64','-64','63.875';'RLR_OBJ24_Track_Age','333','8','BE','unsigned','Standard','0','1','0','0','255';'RLR_OBJ24_Track_ID','169','7','BE','unsigned','Standard','0','1','0','0','127';'RLR_OBJ24_Type','182','3','BE','unsigned','Standard','0','1','0','0','7';'RLR_OBJ24_Width','187','11','BE','unsigned','Standard','0','0.01','0','0','12';'RLR_RollingCounter_0x1D1','360','4','BE','unsigned','Standard','0','1','0','0','15'}  IDPort=off  TimestampPort=off  ErrorPort=off  RemotePort=off  LengthPort=off  StatusPort=off  BRSPort=off  ESIPort=off  DLCPort=off  ApplyMinMax=off
      settings: SourceProductBaseCode=ME,XP,VN  DataFormat=CANdb specified signals
  Data Type Conversion1 : DataTypeConversion  OutDataTypeStr=uint16  SaturateOnIntegerOverflow=off  RndMeth=Floor
  Data Type Conversion{4,8..10,13,19..20,24,28..30,33,39..40,42} (15 alike) : DataTypeConversion  OutDataTypeStr=int8  SaturateOnIntegerOverflow=off  RndMeth=Floor
  Data Type Conversion{2..3,5..7,11..12,14..17,21..23,25..27,31..32,34..37,41} (24 alike) : DataTypeConversion  OutDataTypeStr=single  SaturateOnIntegerOverflow=off  RndMeth=Floor
  Data Type Conversion18 : DataTypeConversion  OutDataTypeStr=uint8  SaturateOnIntegerOverflow=off  RndMeth=Floor
  Data Type Conversion38 : DataTypeConversion  OutDataTypeStr=uint8  SaturateOnIntegerOverflow=off  RndMeth=Floor
  SRR_ADCU_RLR_OBJPos12_0x1D1FromOutData : Outport  OutDataTypeStr=Bus:SRR_ADCU_RLR_OBJPos12_0x1D1
  wires:
  CAN FD Unpack/1 -> Data Type Conversion1/1
  CAN FD Unpack/2 -> Data Type Conversion2/1
  CAN FD Unpack/3 -> Data Type Conversion3/1
  CAN FD Unpack/4 -> Data Type Conversion4/1
  CAN FD Unpack/5 -> Data Type Conversion5/1
  CAN FD Unpack/6 -> Data Type Conversion6/1
  CAN FD Unpack/7 -> Data Type Conversion7/1
  CAN FD Unpack/8 -> Data Type Conversion8/1
  CAN FD Unpack/9 -> Data Type Conversion9/1
  CAN FD Unpack/10 -> Data Type Conversion10/1
  CAN FD Unpack/11 -> Data Type Conversion11/1
  CAN FD Unpack/12 -> Data Type Conversion12/1
  CAN FD Unpack/13 -> Data Type Conversion13/1
  CAN FD Unpack/14 -> Data Type Conversion14/1
  CAN FD Unpack/15 -> Data Type Conversion15/1
  CAN FD Unpack/16 -> Data Type Conversion16/1
  CAN FD Unpack/17 -> Data Type Conversion17/1
  CAN FD Unpack/18 -> Data Type Conversion18/1
  CAN FD Unpack/19 -> Data Type Conversion19/1
  CAN FD Unpack/20 -> Data Type Conversion20/1
  CAN FD Unpack/21 -> Data Type Conversion21/1
  CAN FD Unpack/22 -> Data Type Conversion22/1
  CAN FD Unpack/23 -> Data Type Conversion23/1
  CAN FD Unpack/24 -> Data Type Conversion24/1
  CAN FD Unpack/25 -> Data Type Conversion25/1
  CAN FD Unpack/26 -> Data Type Conversion26/1
  CAN FD Unpack/27 -> Data Type Conversion27/1
  CAN FD Unpack/28 -> Data Type Conversion28/1
  CAN FD Unpack/29 -> Data Type Conversion29/1
  CAN FD Unpack/30 -> Data Type Conversion30/1
  CAN FD Unpack/31 -> Data Type Conversion31/1
  CAN FD Unpack/32 -> Data Type Conversion32/1
  CAN FD Unpack/33 -> Data Type Conversion33/1
  CAN FD Unpack/34 -> Data Type Conversion34/1
  CAN FD Unpack/35 -> Data Type Conversion35/1
  CAN FD Unpack/36 -> Data Type Conversion36/1
  CAN FD Unpack/37 -> Data Type Conversion37/1
  CAN FD Unpack/38 -> Data Type Conversion38/1
  CAN FD Unpack/39 -> Data Type Conversion39/1
  CAN FD Unpack/40 -> Data Type Conversion40/1
  CAN FD Unpack/41 -> Data Type Conversion41/1
  CAN FD Unpack/42 -> Data Type Conversion42/1
  Data Type Conversion1/1 -> Bus Creator/1  "RLR_CRCCheck_0x1D1"
  Data Type Conversion2/1 -> Bus Creator/2  "RLR_OBJ23_Dx"
  Data Type Conversion3/1 -> Bus Creator/3  "RLR_OBJ23_Dy"
  Data Type Conversion4/1 -> Bus Creator/4  "RLR_OBJ23_ExistProb"
  Data Type Conversion5/1 -> Bus Creator/5  "RLR_OBJ23_HeadingAngle"
  Data Type Conversion6/1 -> Bus Creator/6  "RLR_OBJ23_Height"
  Data Type Conversion7/1 -> Bus Creator/7  "RLR_OBJ23_Length"
  Data Type Conversion8/1 -> Bus Creator/8  "RLR_OBJ23_Measured"
  Data Type Conversion9/1 -> Bus Creator/9  "RLR_OBJ23_Motion_Status"
  Data Type Conversion10/1 -> Bus Creator/10  "RLR_OBJ23_ObstacleProb"
  Data Type Conversion11/1 -> Bus Creator/11  "RLR_OBJ23_RefPointDx"
  Data Type Conversion12/1 -> Bus Creator/12  "RLR_OBJ23_RefPointDy"
  Data Type Conversion13/1 -> Bus Creator/13  "RLR_OBJ23_RefPointLoc"
  Data Type Conversion14/1 -> Bus Creator/14  "RLR_OBJ23_RelAx"
  Data Type Conversion15/1 -> Bus Creator/15  "RLR_OBJ23_RelAy"
  Data Type Conversion16/1 -> Bus Creator/16  "RLR_OBJ23_RelVx"
  Data Type Conversion17/1 -> Bus Creator/17  "RLR_OBJ23_RelVy"
  Data Type Conversion18/1 -> Bus Creator/18  "RLR_OBJ23_Track_Age"
  Data Type Conversion19/1 -> Bus Creator/19  "RLR_OBJ23_Track_ID"
  Data Type Conversion20/1 -> Bus Creator/20  "RLR_OBJ23_Type"
  Data Type Conversion21/1 -> Bus Creator/21  "RLR_OBJ23_Width"
  Data Type Conversion22/1 -> Bus Creator/22  "RLR_OBJ24_Dx"
  Data Type Conversion23/1 -> Bus Creator/23  "RLR_OBJ24_Dy"
  Data Type Conversion24/1 -> Bus Creator/24  "RLR_OBJ24_ExistProb"
  Data Type Conversion25/1 -> Bus Creator/25  "RLR_OBJ24_HeadingAngle"
  Data Type Conversion26/1 -> Bus Creator/26  "RLR_OBJ24_Height"
  Data Type Conversion27/1 -> Bus Creator/27  "RLR_OBJ24_Length"
  Data Type Conversion28/1 -> Bus Creator/28  "RLR_OBJ24_Measured"
  Data Type Conversion29/1 -> Bus Creator/29  "RLR_OBJ24_Motion_Status"
  Data Type Conversion30/1 -> Bus Creator/30  "RLR_OBJ24_ObstacleProb"
  Data Type Conversion31/1 -> Bus Creator/31  "RLR_OBJ24_RefPointDx"
  Data Type Conversion32/1 -> Bus Creator/32  "RLR_OBJ24_RefPointDy"
  Data Type Conversion33/1 -> Bus Creator/33  "RLR_OBJ24_RefPointLoc"
  Data Type Conversion34/1 -> Bus Creator/34  "RLR_OBJ24_RelAx"
  Data Type Conversion35/1 -> Bus Creator/35  "RLR_OBJ24_RelAy"
  Data Type Conversion36/1 -> Bus Creator/36  "RLR_OBJ24_RelVx"
  Data Type Conversion37/1 -> Bus Creator/37  "RLR_OBJ24_RelVy"
  Data Type Conversion38/1 -> Bus Creator/38  "RLR_OBJ24_Track_Age"
  Data Type Conversion39/1 -> Bus Creator/39  "RLR_OBJ24_Track_ID"
  Data Type Conversion40/1 -> Bus Creator/40  "RLR_OBJ24_Type"
  Data Type Conversion41/1 -> Bus Creator/41  "RLR_OBJ24_Width"
  Data Type Conversion42/1 -> Bus Creator/42  "RLR_RollingCounter_0x1D1"
  Bus Creator/1 -> SRR_ADCU_RLR_OBJPos12_0x1D1FromOutData/1  "SRR_ADCU_RLR_OBJPos12_0x1D1FromOutData"
  SRR_ADCU_RLR_OBJPos12_0x1D1FromInData/1 -> CAN FD Unpack/1  "SRR_ADCU_RLR_OBJPos12_0x1D1FromInData"
